simulink model "HSat_orbit_merged_maria"  (R2023b)
settings: Solver=FixedStepAuto  StartTime=0  StopTime=86400*900  MaxStep=3600  RelTol=1e-3  EnableMultiTasking=on
values from neighbouring files (symbols this model uses):
  alpha_acc = sqrt(0.7)    [HSat_op_setup_merged_maria.m]    (also in init_orbit_analysis_with_drag_loss.m)
  ext_ENV_G = 6.674e-11    [HSat_op_setup.m]    (also in HSat_op_setup_merged_maria.m)
  ext_ENV_muEarth = 3.986005e14    (= 398600500000000)    [GEO_insertion_setup.m]    (also in HSat_op_setup.m; HSat_op_setup_merged_maria.m; init_orbit_analysis_with_drag_loss.m)
  ext_ENV_Re = 6.37813700*10^6    (= 6378137)    [HSat_op_setup.m]    (also in HSat_op_setup_merged_maria.m)
  ext_EOR_atmosphere_end = 1000e3    (= 1000000)    [HSat_op_setup.m]    (also in HSat_op_setup_merged_maria.m)
  ext_EOR_perigeeraise_end = 600e3    (= 600000)    [HSat_op_setup.m]    (also in HSat_op_setup_merged_maria.m)
  ext_Main_initDate_IC_T = sim_start    [HSat_op_setup.m]    (also in HSat_op_setup_merged_maria.m)
  ext_SC_activecorr_COE_ECI = [1, 1, 1, 0, 0, 0, 0, 0 ]    [HSat_op_setup.m]    (also in HSat_op_setup_merged_maria.m)
  ext_SC_balanced_COE_ECI = [ .500    0.70    1.100 1 1]    [HSat_op_setup.m]    (also in HSat_op_setup_merged_maria.m = [ 0.10 2.10 1.40    1.0000    1.0000]; launch_settings.m)
  ext_SC_cutofferror_COE_ECI = [150e3, .01, 0.1*pi/180, .1*pi/180,.1*pi/180, 0, 0, 0]    [HSat_op_setup.m]    (also in HSat_op_setup_merged_maria.m)
  ext_SC_init_COE_ECI = [a0,ecc0,i0,an0,ap0,tran0,eccan0,ma0]    [HSat_op_setup.m]    (also in HSat_op_setup_merged_maria.m)
  ext_SC_target_COE_ECI = [a1,ecc1,i1,an1,ap1,tran1,eccan1,ma1]    [HSat_op_setup.m]    (also in HSat_op_setup_merged_maria.m)
  ext_SC_target_lambda = 67*pi/180    (= 1.16937059884)    [HSat_op_setup.m]    (also in HSat_op_setup_merged_maria.m)
  flip_timer = 2*60*60    (= 7200)    [HSat_op_setup_merged_maria.m]
  P_solar = 4.56e-6    (= 4.56e-06)    [HSat_op_setup_merged_maria.m]    (also in init_orbit_analysis_with_drag_loss.m)
  sim_SC_init_CoG_EOR_dry = [-0.00448 0.00106 0.46931]    [HSat_op_setup.m]    (also in HSat_op_setup_merged_maria.m)
  sim_SC_init_CoG_propellant = [0 0 0.24758]    [HSat_op_setup.m]    (also in HSat_op_setup_merged_maria.m)
  sim_SC_init_dry_mass = sim_SC_init_wet_mass-sim_SC_init_propellant_mass    (= 727)    [HSat_op_setup.m]    (also in HSat_op_setup_merged_maria.m = 813.7)
  sim_SC_init_MoI_EOR_wet = [ ... (first row only)    [HSat_op_setup.m]    (also in HSat_op_setup_merged_maria.m; init_orbit_analysis_with_drag_loss.m)
  sim_SC_init_wet_mass = 750    [HSat_op_setup.m]    (also in HSat_op_setup_merged_maria.m)
  sim_thrust_force = [ ... (first row only)    [HSat_op_setup.m]    (also in HSat_op_setup_merged_maria.m)
  sim_thrust_massflow = [ ... (first row only)    [HSat_op_setup.m]    (also in HSat_op_setup_merged_maria.m)
  sim_thrust_vector = [ ... (first row only)    [HSat_op_setup.m]    (also in HSat_op_setup_merged_maria.m)
  sim_thruster_position = [ ... (first row only)    [HSat_op_setup.m]    (also in HSat_op_setup_merged_maria.m)
  sim_ts_save = 60    [HSat_op_setup.m]    (also in HSat_op_setup_merged_maria.m)
  sun_pointing_SA = 0    [HSat_op_setup_merged_maria.m]    (also in init_orbit_analysis_with_drag_loss.m)
  third_body_jupiter = 1    [HSat_op_setup.m]    (also in HSat_op_setup_merged_maria.m)
  third_body_moon = 1    [HSat_op_setup.m]    (also in HSat_op_setup_merged_maria.m)
  third_body_sun = 1    [HSat_op_setup.m]    (also in HSat_op_setup_merged_maria.m)
libraries: aerolibutil x59, simulink x18, matrix_library x16, Toolbox x10, sharedtransform x9, sharedutil x5, aerolibatmos2 x1, simulink_extras x1
(part 5 of 8)

== system HSat_orbit_merged_maria/Subsystem1/control/EORattitude/Subsystem4/Attitude for OR thrusters/Subsystem ==
  EORthrustSCB : Inport
  Create 3x3 Matrix : sharedutil/Create 3x3 Matrix  aMode=aMode
      settings: LibrarySourceBlock=aerolibutil/Create 3x3 Matrix
  Demux : Demux  Outputs=3
  Demux1 : Demux  Outputs=3
  Demux2 : Demux  Outputs=3
  Direction Cosine Matrix to Quaternions : sharedtransform/Direction Cosine Matrix  to Quaternions  aMode=0  action=None  tolerance=eps(2)
      settings: LibrarySourceBlock=|
      | aerolibtransform2/Direction Cosine Matrix
      | to Quaternions
  Quaternion Inverse : aerolibutil/Quaternion Inverse
  VecNormalize4 : Subsystem
      mask Display: disp('u/||u||')
  Zeci x Reci : Subsystem  mask(Cross Product){}
      mask help: Calculates the cross product of two 3x1 vectors.
      mask Help:
      | <p>This block calculates the cross product of two 3x1 vectors, ie.</p>
      | 
      | <ul>C(1) = A(2)*B(3) - A(3)*B(2)</ul>
      | <ul>C(2) = A(3)*B(1) - A(1)*B(3)</ul>
      | <ul>C(3) = A(1)*B(2) - A(2)*B(1)</ul>
      | 
      | <p>The block inputs and output contain more than one signal as described below.</p>
      | 
      | <p><H4>Block Vector Input 1 - A</H4>
      | <ul>
      | <li>A(1)</li>
      | <li>A(2)</li>
      | <li>A(3)</li>
      | </ul>
      | </p>
      | 
      | <p><H4>Block Vector Input 2 - B</H4>
      | <ul>
      | <li>B(1)</li>
      | <li>B(2)</li>
      | <li>B(3)</li>
      | </ul>
      | </p>
      | 
      | <p><H4>Block Vector Output - Cross Product (AxB)</H4>
      | <ul>
      | <li>C(1)</li>
      | <li>C(2)</li>
      | <li>C(3)</li>
      | </ul>
      | </p>
      mask Display: disp('Cross\nProduct')
  Zeci x Reci1 : Subsystem  mask(Cross Product){}
      mask help: Calculates the cross product of two 3x1 vectors.
      mask Help:
      | <p>This block calculates the cross product of two 3x1 vectors, ie.</p>
      | 
      | <ul>C(1) = A(2)*B(3) - A(3)*B(2)</ul>
      | <ul>C(2) = A(3)*B(1) - A(1)*B(3)</ul>
      | <ul>C(3) = A(1)*B(2) - A(2)*B(1)</ul>
      | 
      | <p>The block inputs and output contain more than one signal as described below.</p>
      | 
      | <p><H4>Block Vector Input 1 - A</H4>
      | <ul>
      | <li>A(1)</li>
      | <li>A(2)</li>
      | <li>A(3)</li>
      | </ul>
      | </p>
      | 
      | <p><H4>Block Vector Input 2 - B</H4>
      | <ul>
      | <li>B(1)</li>
      | <li>B(2)</li>
      | <li>B(3)</li>
      | </ul>
      | </p>
      | 
      | <p><H4>Block Vector Output - Cross Product (AxB)</H4>
      | <ul>
      | <li>C(1)</li>
      | <li>C(2)</li>
      | <li>C(3)</li>
      | </ul>
      | </p>
      mask Display: disp('Cross\nProduct')
  yscbSCB : Constant  Value=[0 1 0]
  qscbp2scb : Outport
  wires:
  Direction Cosine Matrix to Quaternions/1 -> Quaternion Inverse/1  "qscbp2scb"
  Demux2/3 -> Create 3x3 Matrix/9
  Demux2/1 -> Create 3x3 Matrix/7
  Demux/1 -> Create 3x3 Matrix/1
  Demux1/2 -> Create 3x3 Matrix/5
  EORthrustSCB/1 -> VecNormalize4/1(In1)
  Demux2/2 -> Create 3x3 Matrix/8
  Demux/3 -> Create 3x3 Matrix/3
  Zeci x Reci/1(c(1) c(2) c(3)) -> Zeci x Reci1/2(b(1) b(2) b(3)), Demux/1  "xscbpSCB"
  Demux/2 -> Create 3x3 Matrix/2
  Create 3x3 Matrix/1 -> Direction Cosine Matrix to Quaternions/1
  Zeci x Reci1/1(c(1) c(2) c(3)) -> Demux1/1  "yscbpSCB"
  Demux1/3 -> Create 3x3 Matrix/6
  Demux1/1 -> Create 3x3 Matrix/4
  yscbSCB/1 -> Zeci x Reci/1(a(1) a(2) a(3))
  VecNormalize4/1(Out1) -> Demux2/1, Zeci x Reci1/1(a(1) a(2) a(3)), Zeci x Reci/2(b(1) b(2) b(3))  "zscbpSCB"
  Quaternion Inverse/1 -> qscbp2scb/1

== system HSat_orbit_merged_maria/Subsystem1/control/EORattitude/Subsystem4/Attitude for OR thrusters/q_scb_calc ==
  EORthrustECI : Inport
  sunvECI : Inport  Port=2
  Direction Cosine Matrix to Quaternions : sharedtransform/Direction Cosine Matrix  to Quaternions  aMode=0  action=None  tolerance=eps(2)
      settings: LibrarySourceBlock=|
      | aerolibtransform2/Direction Cosine Matrix
      | to Quaternions
  Matrix Concatenate : Concatenate  NumInputs=3  Mode=Multidimensional array
  Reshape1 : Reshape  OutputDimensionality=Row vector (2-D)
  Reshape2 : Reshape  OutputDimensionality=Row vector (2-D)
  Reshape3 : Reshape  OutputDimensionality=Row vector (2-D)
  VecNormalize : Subsystem
      mask Display: disp('u/||u||')
  VecNormalize1 : Subsystem
      mask Display: disp('u/||u||')
  VecNormalize2 : Subsystem
      mask Display: disp('u/||u||')
  VecNormalize3 : Subsystem
      mask Display: disp('u/||u||')
  Yscb x Zscb : Subsystem  mask(Cross Product){}
      mask help: Calculates the cross product of two 3x1 vectors.
      mask Help:
      | <p>This block calculates the cross product of two 3x1 vectors, ie.</p>
      | 
      | <ul>C(1) = A(2)*B(3) - A(3)*B(2)</ul>
      | <ul>C(2) = A(3)*B(1) - A(1)*B(3)</ul>
      | <ul>C(3) = A(1)*B(2) - A(2)*B(1)</ul>
      | 
      | <p>The block inputs and output contain more than one signal as described below.</p>
      | 
      | <p><H4>Block Vector Input 1 - A</H4>
      | <ul>
      | <li>A(1)</li>
      | <li>A(2)</li>
      | <li>A(3)</li>
      | </ul>
      | </p>
      | 
      | <p><H4>Block Vector Input 2 - B</H4>
      | <ul>
      | <li>B(1)</li>
      | <li>B(2)</li>
      | <li>B(3)</li>
      | </ul>
      | </p>
      | 
      | <p><H4>Block Vector Output - Cross Product (AxB)</H4>
      | <ul>
      | <li>C(1)</li>
      | <li>C(2)</li>
      | <li>C(3)</li>
      | </ul>
      | </p>
      mask Display: disp('Cross\nProduct')
  Zeci x Reci : Subsystem  mask(Cross Product){}
      mask help: Calculates the cross product of two 3x1 vectors.
      mask Help:
      | <p>This block calculates the cross product of two 3x1 vectors, ie.</p>
      | 
      | <ul>C(1) = A(2)*B(3) - A(3)*B(2)</ul>
      | <ul>C(2) = A(3)*B(1) - A(1)*B(3)</ul>
      | <ul>C(3) = A(1)*B(2) - A(2)*B(1)</ul>
      | 
      | <p>The block inputs and output contain more than one signal as described below.</p>
      | 
      | <p><H4>Block Vector Input 1 - A</H4>
      | <ul>
      | <li>A(1)</li>
      | <li>A(2)</li>
      | <li>A(3)</li>
      | </ul>
      | </p>
      | 
      | <p><H4>Block Vector Input 2 - B</H4>
      | <ul>
      | <li>B(1)</li>
      | <li>B(2)</li>
      | <li>B(3)</li>
      | </ul>
      | </p>
      | 
      | <p><H4>Block Vector Output - Cross Product (AxB)</H4>
      | <ul>
      | <li>C(1)</li>
      | <li>C(2)</li>
      | <li>C(3)</li>
      | </ul>
      | </p>
      mask Display: disp('Cross\nProduct')
  qECI2scbp : Outport  InitialOutput=0
  wires:
  Zeci x Reci/1(c(1) c(2) c(3)) -> VecNormalize3/1(In1)  "Y"
  VecNormalize1/1(Out1) -> Yscb x Zscb/2(b(1) b(2) b(3)), Reshape3/1, Zeci x Reci/2(b(1) b(2) b(3))  "Zscbp"
  Direction Cosine Matrix to Quaternions/1 -> qECI2scbp/1
  EORthrustECI/1 -> VecNormalize1/1(In1)
  VecNormalize3/1(Out1) -> Reshape1/1, Yscb x Zscb/1(a(1) a(2) a(3))  "Yscbp"
  Yscb x Zscb/1(c(1) c(2) c(3)) -> VecNormalize/1(In1)
  sunvECI/1 -> VecNormalize2/1(In1)
  Reshape1/1 -> Matrix Concatenate/2
  Reshape3/1 -> Matrix Concatenate/3
  Reshape2/1 -> Matrix Concatenate/1
  VecNormalize/1(Out1) -> Reshape2/1  "Xscbp"
  VecNormalize2/1(Out1) -> Zeci x Reci/1(a(1) a(2) a(3))
  Matrix Concatenate/1 -> Direction Cosine Matrix to Quaternions/1

== system HSat_orbit_merged_maria/Subsystem1/control/EORattitude/Subsystem4/Attitude for SK unloading/Subsystem ==
  SKtorqueSCB : Inport
  Create 3x3 Matrix : sharedutil/Create 3x3 Matrix  aMode=aMode
      settings: LibrarySourceBlock=aerolibutil/Create 3x3 Matrix
  Demux : Demux  Outputs=3
  Demux1 : Demux  Outputs=3
  Demux2 : Demux  Outputs=3
  Direction Cosine Matrix to Quaternions : sharedtransform/Direction Cosine Matrix  to Quaternions  aMode=0  action=None  tolerance=eps(2)
      settings: LibrarySourceBlock=|
      | aerolibtransform2/Direction Cosine Matrix
      | to Quaternions
  Quaternion Inverse : aerolibutil/Quaternion Inverse
  VecNormalize4 : Subsystem
      mask Display: disp('u/||u||')
  Zeci x Reci : Subsystem  mask(Cross Product){}
      mask help: Calculates the cross product of two 3x1 vectors.
      mask Help:
      | <p>This block calculates the cross product of two 3x1 vectors, ie.</p>
      | 
      | <ul>C(1) = A(2)*B(3) - A(3)*B(2)</ul>
      | <ul>C(2) = A(3)*B(1) - A(1)*B(3)</ul>
      | <ul>C(3) = A(1)*B(2) - A(2)*B(1)</ul>
      | 
      | <p>The block inputs and output contain more than one signal as described below.</p>
      | 
      | <p><H4>Block Vector Input 1 - A</H4>
      | <ul>
      | <li>A(1)</li>
      | <li>A(2)</li>
      | <li>A(3)</li>
      | </ul>
      | </p>
      | 
      | <p><H4>Block Vector Input 2 - B</H4>
      | <ul>
      | <li>B(1)</li>
      | <li>B(2)</li>
      | <li>B(3)</li>
      | </ul>
      | </p>
      | 
      | <p><H4>Block Vector Output - Cross Product (AxB)</H4>
      | <ul>
      | <li>C(1)</li>
      | <li>C(2)</li>
      | <li>C(3)</li>
      | </ul>
      | </p>
      mask Display: disp('Cross\nProduct')
  Zeci x Reci1 : Subsystem  mask(Cross Product){}
      mask help: Calculates the cross product of two 3x1 vectors.
      mask Help:
      | <p>This block calculates the cross product of two 3x1 vectors, ie.</p>
      | 
      | <ul>C(1) = A(2)*B(3) - A(3)*B(2)</ul>
      | <ul>C(2) = A(3)*B(1) - A(1)*B(3)</ul>
      | <ul>C(3) = A(1)*B(2) - A(2)*B(1)</ul>
      | 
      | <p>The block inputs and output contain more than one signal as described below.</p>
      | 
      | <p><H4>Block Vector Input 1 - A</H4>
      | <ul>
      | <li>A(1)</li>
      | <li>A(2)</li>
      | <li>A(3)</li>
      | </ul>
      | </p>
      | 
      | <p><H4>Block Vector Input 2 - B</H4>
      | <ul>
      | <li>B(1)</li>
      | <li>B(2)</li>
      | <li>B(3)</li>
      | </ul>
      | </p>
      | 
      | <p><H4>Block Vector Output - Cross Product (AxB)</H4>
      | <ul>
      | <li>C(1)</li>
      | <li>C(2)</li>
      | <li>C(3)</li>
      | </ul>
      | </p>
      mask Display: disp('Cross\nProduct')
  yscbSCB : Constant  Value=[0 1 0]
  qscbp2scb : Outport
  wires:
  Direction Cosine Matrix to Quaternions/1 -> Quaternion Inverse/1  "qscbp2scb"
  Demux2/3 -> Create 3x3 Matrix/9
  Demux2/1 -> Create 3x3 Matrix/7
  Demux/1 -> Create 3x3 Matrix/1
  Demux1/2 -> Create 3x3 Matrix/5
  SKtorqueSCB/1 -> VecNormalize4/1(In1)
  Demux2/2 -> Create 3x3 Matrix/8
  Demux/3 -> Create 3x3 Matrix/3
  Zeci x Reci/1(c(1) c(2) c(3)) -> Zeci x Reci1/2(b(1) b(2) b(3)), Demux/1  "xscbpSCB"
  Demux/2 -> Create 3x3 Matrix/2
  Create 3x3 Matrix/1 -> Direction Cosine Matrix to Quaternions/1
  Zeci x Reci1/1(c(1) c(2) c(3)) -> Demux1/1  "yscbpSCB"
  Demux1/3 -> Create 3x3 Matrix/6
  Demux1/1 -> Create 3x3 Matrix/4
  yscbSCB/1 -> Zeci x Reci/1(a(1) a(2) a(3))
  VecNormalize4/1(Out1) -> Demux2/1, Zeci x Reci1/1(a(1) a(2) a(3)), Zeci x Reci/2(b(1) b(2) b(3))  "zscbpSCB"
  Quaternion Inverse/1 -> qscbp2scb/1

== system HSat_orbit_merged_maria/Subsystem1/control/EORattitude/Subsystem4/Attitude for SK unloading/VecNormalize ==
  In1 : Inport
  Constant : Constant
  Demux : Demux  Outputs=[-1 1]
  Divide : Product  Inputs=*/  OutDataTypeStr=double
  Ground : Ground
  Math Function : Math  Operator=square  SignedPower=on
  Math Function1 : Math  Operator=sqrt  SignedPower=on
  Mux : Mux  Inputs=2
  Mux1 : Mux  Inputs=2
  Product : Product  RndMeth=Zero
  Sum of Elements : Sum  Inputs=+
  Switch : Switch  Criteria=u2 > Threshold  Threshold=eps  SaturateOnIntegerOverflow=off  InputSameDT=off
  Out1 : Outport  VectorParamsAs1DForOutWhenUnconnected=off
  wires:
  Math Function/1 -> Sum of Elements/1
  Demux/1 -> Divide/1
  Constant/1 -> Mux1/2
  Mux1/1 -> Switch/3
  Divide/1 -> Out1/1
  Switch/1 -> Demux/1
  Mux/1 -> Switch/1
  Demux/2 -> Divide/2
  Product/1 -> Mux1/1
  In1/1 -> Product/1, Math Function/1, Mux/1
  Ground/1 -> Product/2
  Sum of Elements/1 -> Math Function1/1
  Math Function1/1 -> Mux/2, Switch/2

== system HSat_orbit_merged_maria/Subsystem1/control/EORattitude/Subsystem4/Attitude for SK unloading/VecNormalize1 ==
  In1 : Inport
  Constant : Constant
  Demux : Demux  Outputs=[-1 1]
  Divide : Product  Inputs=*/  OutDataTypeStr=double
  Ground : Ground
  Math Function : Math  Operator=square  SignedPower=on
  Math Function1 : Math  Operator=sqrt  SignedPower=on
  Mux : Mux  Inputs=2
  Mux1 : Mux  Inputs=2
  Product : Product  RndMeth=Zero
  Sum of Elements : Sum  Inputs=+
  Switch : Switch  Criteria=u2 > Threshold  Threshold=eps  SaturateOnIntegerOverflow=off  InputSameDT=off
  Out1 : Outport  VectorParamsAs1DForOutWhenUnconnected=off
  wires:
  Math Function/1 -> Sum of Elements/1
  Demux/1 -> Divide/1
  Constant/1 -> Mux1/2
  Mux1/1 -> Switch/3
  Divide/1 -> Out1/1
  Switch/1 -> Demux/1
  Mux/1 -> Switch/1
  Demux/2 -> Divide/2
  Product/1 -> Mux1/1
  In1/1 -> Product/1, Math Function/1, Mux/1
  Ground/1 -> Product/2
  Sum of Elements/1 -> Math Function1/1
  Math Function1/1 -> Mux/2, Switch/2

== system HSat_orbit_merged_maria/Subsystem1/control/EORattitude/Subsystem4/Attitude for SK unloading/VecNormalize2 ==
  In1 : Inport
  Constant : Constant
  Demux : Demux  Outputs=[-1 1]
  Divide : Product  Inputs=*/  OutDataTypeStr=double
  Ground : Ground
  Math Function : Math  Operator=square  SignedPower=on
  Math Function1 : Math  Operator=sqrt  SignedPower=on
  Mux : Mux  Inputs=2
  Mux1 : Mux  Inputs=2
  Product : Product  RndMeth=Zero
  Sum of Elements : Sum  Inputs=+
  Switch : Switch  Criteria=u2 > Threshold  Threshold=eps  SaturateOnIntegerOverflow=off  InputSameDT=off
  Out1 : Outport  VectorParamsAs1DForOutWhenUnconnected=off
  wires:
  Math Function/1 -> Sum of Elements/1
  Demux/1 -> Divide/1
  Constant/1 -> Mux1/2
  Mux1/1 -> Switch/3
  Divide/1 -> Out1/1
  Switch/1 -> Demux/1
  Mux/1 -> Switch/1
  Demux/2 -> Divide/2
  Product/1 -> Mux1/1
  In1/1 -> Product/1, Math Function/1, Mux/1
  Ground/1 -> Product/2
  Sum of Elements/1 -> Math Function1/1
  Math Function1/1 -> Mux/2, Switch/2

== system HSat_orbit_merged_maria/Subsystem1/control/EORattitude/Subsystem4/Attitude for SK unloading/VecNormalize3 ==
  In1 : Inport
  Constant : Constant
  Demux : Demux  Outputs=[-1 1]
  Divide : Product  Inputs=*/  OutDataTypeStr=double
  Ground : Ground
  Math Function : Math  Operator=square  SignedPower=on
  Math Function1 : Math  Operator=sqrt  SignedPower=on
  Mux : Mux  Inputs=2
  Mux1 : Mux  Inputs=2
  Product : Product  RndMeth=Zero
  Sum of Elements : Sum  Inputs=+
  Switch : Switch  Criteria=u2 > Threshold  Threshold=eps  SaturateOnIntegerOverflow=off  InputSameDT=off
  Out1 : Outport  VectorParamsAs1DForOutWhenUnconnected=off
  wires:
  Math Function/1 -> Sum of Elements/1
  Demux/1 -> Divide/1
  Constant/1 -> Mux1/2
  Mux1/1 -> Switch/3
  Divide/1 -> Out1/1
  Switch/1 -> Demux/1
  Mux/1 -> Switch/1
  Demux/2 -> Divide/2
  Product/1 -> Mux1/1
  In1/1 -> Product/1, Math Function/1, Mux/1
  Ground/1 -> Product/2
  Sum of Elements/1 -> Math Function1/1
  Math Function1/1 -> Mux/2, Switch/2

== system HSat_orbit_merged_maria/Subsystem1/control/EORattitude/Subsystem4/Attitude for SK unloading/Yscb x Zscb ==
  a(1) a(2) a(3) : Inport
  b(1) b(2) b(3) : Inport  Port=2
  Product : Product  InputSameDT=on  SaturateOnIntegerOverflow=on  OutDataTypeStr=Inherit: Same as first input
  Product1 : Product  InputSameDT=on  SaturateOnIntegerOverflow=on  OutDataTypeStr=Inherit: Same as first input
  Selector : Selector  InputPortWidth=3  IndexOptions=Index vector (dialog)  Indices=[2 3 1]  OutputSizes=1
  Selector1 : Selector  InputPortWidth=3  IndexOptions=Index vector (dialog)  Indices=[3 1 2]  OutputSizes=1
  Selector2 : Selector  InputPortWidth=3  IndexOptions=Index vector (dialog)  Indices=[2 3 1]  OutputSizes=1
  Selector3 : Selector  InputPortWidth=3  IndexOptions=Index vector (dialog)  Indices=[3 1 2]  OutputSizes=1
  Sum : Sum  Inputs=+|-  InputSameDT=on  SaturateOnIntegerOverflow=on  OutDataTypeStr=Inherit: Same as first input
  c(1) c(2) c(3) : Outport  InitialOutput=0
  wires:
  Sum/1 -> c(1) c(2) c(3)/1
  b(1) b(2) b(3)/1 -> Selector1/1, Selector2/1
  Selector/1 -> Product/1
  a(1) a(2) a(3)/1 -> Selector/1, Selector3/1
  Product/1 -> Sum/1
  Selector1/1 -> Product/2
  Product1/1 -> Sum/2
  Selector2/1 -> Product1/2
  Selector3/1 -> Product1/1

== system HSat_orbit_merged_maria/Subsystem1/control/EORattitude/Subsystem4/Attitude for SK unloading/Zeci x Reci ==
  a(1) a(2) a(3) : Inport
  b(1) b(2) b(3) : Inport  Port=2
  Product : Product  InputSameDT=on  SaturateOnIntegerOverflow=on  OutDataTypeStr=Inherit: Same as first input
  Product1 : Product  InputSameDT=on  SaturateOnIntegerOverflow=on  OutDataTypeStr=Inherit: Same as first input
  Selector : Selector  InputPortWidth=3  IndexOptions=Index vector (dialog)  Indices=[2 3 1]  OutputSizes=1
  Selector1 : Selector  InputPortWidth=3  IndexOptions=Index vector (dialog)  Indices=[3 1 2]  OutputSizes=1
  Selector2 : Selector  InputPortWidth=3  IndexOptions=Index vector (dialog)  Indices=[2 3 1]  OutputSizes=1
  Selector3 : Selector  InputPortWidth=3  IndexOptions=Index vector (dialog)  Indices=[3 1 2]  OutputSizes=1
  Sum : Sum  Inputs=+|-  InputSameDT=on  SaturateOnIntegerOverflow=on  OutDataTypeStr=Inherit: Same as first input
  c(1) c(2) c(3) : Outport  InitialOutput=0
  wires:
  Selector3/1 -> Product1/1
  Selector2/1 -> Product1/2
  Product1/1 -> Sum/2
  Selector1/1 -> Product/2
  Product/1 -> Sum/1
  a(1) a(2) a(3)/1 -> Selector3/1, Selector/1
  Selector/1 -> Product/1
  b(1) b(2) b(3)/1 -> Selector2/1, Selector1/1
  Sum/1 -> c(1) c(2) c(3)/1

== system HSat_orbit_merged_maria/Subsystem1/control/EORattitude/Subsystem4/Subsystem3/Flip satellite based on worst case faior ==
  AmomSCB : Inport
  thrustscb : Inport  Port=2
  Constant : Constant  Value=sim_SC_init_MoI_EOR_wet
  MATLAB Function : MATLAB Function  TreatAsAtomicUnit=on
  Reshape : Reshape  OutputDimensionality=Column vector (2-D)
  Scope : Scope  NumInputPorts=2
  worstRwMom : Outport
  isFlip : Outport  Port=2
  idxMinMom : Outport  Port=3
  wires:
  AmomSCB/1 -> Reshape/1
  thrustscb/1 -> MATLAB Function/2(thrustVect)
  MATLAB Function/1(worstRwMom) -> Scope/1, worstRwMom/1  "worstRwmom"
  MATLAB Function/2(isFlip) -> Scope/2, isFlip/1  "flip"
  MATLAB Function/3(idxMaxMom) -> idxMinMom/1
  Constant/1 -> MATLAB Function/3(scInertia)
  Reshape/1 -> MATLAB Function/1(scMom)

== system HSat_orbit_merged_maria/Subsystem1/control/EORattitude/Subsystem4/Subsystem3/FlipSatellite ==
  AmomSCB : Inport
  EORtorqueSCB : Inport  Port=2
  Compare To Constant : simulink/Logic and Bit Operations/Compare To Constant  relop=>  const=sin((180-70.53)/2*pi/180)*25*.75  OutDataTypeStr=boolean
  Compare To Constant1 : simulink/Logic and Bit Operations/Compare To Constant  relop=>  const=cos(80*pi/180)  OutDataTypeStr=boolean
  Compare To Constant2 : simulink/Logic and Bit Operations/Compare To Constant  relop=>  const=sin((180-70.53)/2*pi/180)*25*.8  OutDataTypeStr=boolean
  Compare To Constant3 : simulink/Logic and Bit Operations/Compare To Constant  relop=>  const=cos(90*pi/180)  OutDataTypeStr=boolean
  Dot Product : DotProduct  OutDataTypeStr=Inherit: Inherit via internal rule
  Dot Product1 : DotProduct  OutDataTypeStr=Inherit: Inherit via internal rule
  Logical Operator : Logic  AllPortsSameDT=off  OutDataTypeStr=boolean
  Logical Operator1 : Logic  AllPortsSameDT=off  OutDataTypeStr=boolean
  Logical Operator2 : Logic  Operator=OR  AllPortsSameDT=off  OutDataTypeStr=boolean
  Logical Operator3 : Logic  Operator=NOT  AllPortsSameDT=off  OutDataTypeStr=boolean
  Reshape1 : Reshape  OutputDimensionality=Row vector (2-D)
  VecNormalize : Subsystem
      mask Display: disp('u/||u||')
  VecNormalize1 : Subsystem
      mask Display: disp('u/||u||')
  FlipSatellite_bool : Outport
  DoAMOM : Outport  Port=2
  NoAMOM : Outport  Port=3
  wires:
  Logical Operator/1 -> Logical Operator2/1
  EORtorqueSCB/1 -> VecNormalize1/1(In1)
  Dot Product/1 -> Compare To Constant2/1, Compare To Constant/1
  Compare To Constant/1 -> Logical Operator/1
  Dot Product1/1 -> Compare To Constant3/1, Compare To Constant1/1
  Compare To Constant1/1 -> Logical Operator/2
  VecNormalize/1(Out1) -> Dot Product/2, Dot Product1/1
  VecNormalize1/1(Out1) -> Dot Product1/2
  Compare To Constant2/1 -> Logical Operator1/1
  Compare To Constant3/1 -> Logical Operator3/1, Logical Operator1/2
  Logical Operator1/1 -> DoAMOM/1, Logical Operator2/2
  Logical Operator2/1 -> FlipSatellite_bool/1
  AmomSCB/1 -> Reshape1/1
  Reshape1/1 -> Dot Product/1, VecNormalize/1(In1)
  Logical Operator3/1 -> NoAMOM/1

== system HSat_orbit_merged_maria/Subsystem1/control/EORattitude/Subsystem4/Subsystem3/Subsystem ==
  note: When FlipNow = 1, FlipPlusMinus changes
      | from 0 -> 1 or 1 -> 0.
      | When FlipNow  = 0, FlipPlusMinus keeps the
      | value it has.
  note: FlipSign
  FlipNow : Inport
  Logical Operator : Logic  Operator=NOT  AllPortsSameDT=off  OutDataTypeStr=boolean
  Switch : Switch  Criteria=u2 > Threshold  SaturateOnIntegerOverflow=off
  Unit Delay : UnitDelay  InitialCondition=false  SampleTime=-1  HasFrameUpgradeWarning=on
  FlipPlusMinus : Outport
  wires:
  FlipNow/1 -> Switch/2
  Logical Operator/1 -> Switch/1
  Switch/1 -> Unit Delay/1, FlipPlusMinus/1
  Unit Delay/1 -> Logical Operator/1, Switch/3

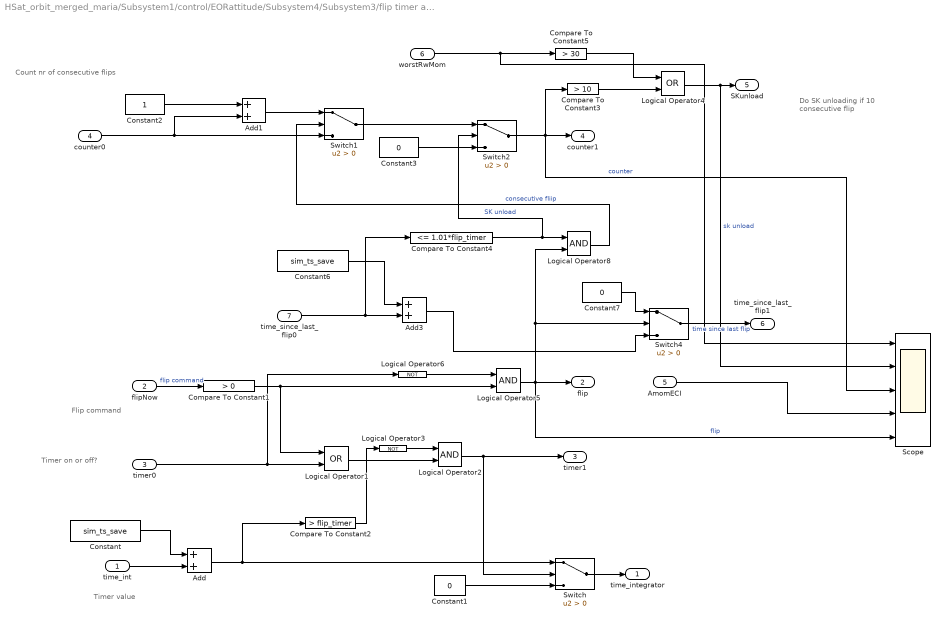
== system HSat_orbit_merged_maria/Subsystem1/control/EORattitude/Subsystem4/Subsystem3/flip timer and SK trigger ==
  note: Timer on or off?
  note: Flip command
  note: Timer value
  note: Count nr of
      | consecutive flips
  note: Do SK unloading
      | if 10 consecutive
      | flip
  time_int : Inport
  flipNow : Inport  Port=2
  timer0 : Inport  Port=3
  counter0 : Inport  Port=4
  AmomECI : Inport  Port=5
  worstRwMom : Inport  Port=6
  time_since_last_flip0 : Inport  Port=7
  Add : Sum
  Add1 : Sum
  Add3 : Sum
  Compare To Constant1 : simulink/Logic and Bit Operations/Compare To Constant  relop=>  const=0  OutDataTypeStr=boolean
  Compare To Constant2 : simulink/Logic and Bit Operations/Compare To Constant  relop=>  const=flip_timer  OutDataTypeStr=boolean
  Compare To Constant3 : simulink/Logic and Bit Operations/Compare To Constant  relop=>  const=10  OutDataTypeStr=boolean
  Compare To Constant4 : simulink/Logic and Bit Operations/Compare To Constant  relop=<=  const=1.01*flip_timer  OutDataTypeStr=boolean
  Compare To Constant5 : simulink/Logic and Bit Operations/Compare To Constant  relop=>  const=30  OutDataTypeStr=boolean
  Constant : Constant  Value=sim_ts_save
  Constant1 : Constant  Value=0
  Constant2 : Constant
  Constant3 : Constant  Value=0
  Constant6 : Constant  Value=sim_ts_save
  Constant7 : Constant  Value=0
  Logical Operator1 : Logic  Operator=OR  AllPortsSameDT=off  OutDataTypeStr=boolean
  Logical Operator2 : Logic  AllPortsSameDT=off  OutDataTypeStr=boolean
  Logical Operator3 : Logic  Operator=NOT  AllPortsSameDT=off  OutDataTypeStr=boolean
  Logical Operator4 : Logic  Operator=OR  AllPortsSameDT=off  OutDataTypeStr=boolean
  Logical Operator5 : Logic  AllPortsSameDT=off  OutDataTypeStr=boolean
  Logical Operator6 : Logic  Operator=NOT  AllPortsSameDT=off  OutDataTypeStr=boolean
  Logical Operator8 : Logic  AllPortsSameDT=off  OutDataTypeStr=boolean
  Scope : Scope  NumInputPorts=5
  Switch{,1..2,4} (4 alike) : Switch  Criteria=u2 > Threshold  SaturateOnIntegerOverflow=off  InputSameDT=off
  time_integrator : Outport
  flip : Outport  Port=2
  timer1 : Outport  Port=3
  counter1 : Outport  Port=4
  SKunload : Outport  Port=5
  time_since_last_flip1 : Outport  Port=6
  wires:
  flipNow/1 -> Compare To Constant1/1  "flip command"
  time_int/1 -> Add/2
  Constant/1 -> Add/1
  Add/1 -> Switch/1, Compare To Constant2/1
  Compare To Constant1/1 -> Logical Operator5/2, Logical Operator1/1
  Compare To Constant2/1 -> Logical Operator3/1
  Logical Operator5/1 -> Switch4/2, Logical Operator8/2, flip/1, Scope/5  "flip"
  Switch/1 -> time_integrator/1
  Constant1/1 -> Switch/3
  Logical Operator1/1 -> Logical Operator2/2
  Logical Operator3/1 -> Logical Operator2/1
  Logical Operator2/1 -> timer1/1, Switch/2
  counter0/1 -> Add1/2, Switch1/3
  Constant2/1 -> Add1/1
  Add1/1 -> Switch1/1
  Switch1/1 -> Switch2/1
  timer0/1 -> Logical Operator6/1, Logical Operator1/2
  Constant3/1 -> Switch2/3
  Switch2/1 -> Scope/3, Compare To Constant3/1, counter1/1  "counter"
  Logical Operator6/1 -> Logical Operator5/1
  AmomECI/1 -> Scope/4
  worstRwMom/1 -> Scope/1, Compare To Constant5/1
  Constant6/1 -> Add3/1
  Add3/1 -> Switch4/3
  Constant7/1 -> Switch4/1
  Switch4/1 -> time_since_last_flip1/1  "time since last flip"
  Compare To Constant4/1 -> Switch2/2, Logical Operator8/1  "SK unload"
  time_since_last_flip0/1 -> Compare To Constant4/1, Add3/2
  Logical Operator8/1 -> Switch1/2  "consecutive fliip"
  Compare To Constant3/1 -> Logical Operator4/2
  Logical Operator4/1 -> Scope/2, SKunload/1  "sk unload"
  Compare To Constant5/1 -> Logical Operator4/1

== system HSat_orbit_merged_maria/Subsystem1/control/EORattitude/Subsystem4/flips around thrust vector/VecNormalize4 ==
  In1 : Inport
  Constant : Constant
  Demux : Demux  Outputs=[-1 1]
  Divide : Product  Inputs=*/  OutDataTypeStr=double
  Ground : Ground
  Math Function : Math  Operator=square  SignedPower=on
  Math Function1 : Math  Operator=sqrt  SignedPower=on
  Mux : Mux  Inputs=2
  Mux1 : Mux  Inputs=2
  Product : Product  RndMeth=Zero
  Sum of Elements : Sum  Inputs=+
  Switch : Switch  Criteria=u2 > Threshold  Threshold=eps  SaturateOnIntegerOverflow=off  InputSameDT=off
  Out1 : Outport  VectorParamsAs1DForOutWhenUnconnected=off
  wires:
  Math Function/1 -> Sum of Elements/1
  Demux/1 -> Divide/1
  Constant/1 -> Mux1/2
  Mux1/1 -> Switch/3
  Divide/1 -> Out1/1
  Switch/1 -> Demux/1
  Mux/1 -> Switch/1
  Demux/2 -> Divide/2
  Product/1 -> Mux1/1
  In1/1 -> Product/1, Math Function/1, Mux/1
  Ground/1 -> Product/2
  Sum of Elements/1 -> Math Function1/1
  Math Function1/1 -> Mux/2, Switch/2

== system HSat_orbit_merged_maria/Subsystem1/control/Subsystem6/Subsystem2/PPU1/VecNormalize1 ==
  In1 : Inport
  Constant : Constant
  Demux : Demux  Outputs=[-1 1]
  Divide : Product  Inputs=*/  OutDataTypeStr=double
  Ground : Ground
  Math Function : Math  Operator=square  SignedPower=on
  Math Function1 : Math  Operator=sqrt  SignedPower=on
  Mux : Mux  Inputs=2
  Mux1 : Mux  Inputs=2
  Product : Product  RndMeth=Zero
  Sum of Elements : Sum  Inputs=+
  Switch : Switch  Criteria=u2 > Threshold  Threshold=eps  SaturateOnIntegerOverflow=off  InputSameDT=off
  Out1 : Outport  VectorParamsAs1DForOutWhenUnconnected=off
  wires:
  Math Function/1 -> Sum of Elements/1
  Demux/1 -> Divide/1
  Constant/1 -> Mux1/2
  Mux1/1 -> Switch/3
  Divide/1 -> Out1/1
  Switch/1 -> Demux/1
  Mux/1 -> Switch/1
  Demux/2 -> Divide/2
  Product/1 -> Mux1/1
  In1/1 -> Product/1, Math Function/1, Mux/1
  Ground/1 -> Product/2
  Sum of Elements/1 -> Math Function1/1
  Math Function1/1 -> Mux/2, Switch/2

== system HSat_orbit_merged_maria/Subsystem1/control/Subsystem6/Subsystem2/PPU1/VecNormalize2 ==
  In1 : Inport
  Constant : Constant
  Demux : Demux  Outputs=[-1 1]
  Divide : Product  Inputs=*/  OutDataTypeStr=double
  Ground : Ground
  Math Function : Math  Operator=square  SignedPower=on
  Math Function1 : Math  Operator=sqrt  SignedPower=on
  Mux : Mux  Inputs=2
  Mux1 : Mux  Inputs=2
  Product : Product  RndMeth=Zero
  Sum of Elements : Sum  Inputs=+
  Switch : Switch  Criteria=u2 > Threshold  Threshold=eps  SaturateOnIntegerOverflow=off  InputSameDT=off
  Out1 : Outport  VectorParamsAs1DForOutWhenUnconnected=off
  wires:
  Math Function/1 -> Sum of Elements/1
  Demux/1 -> Divide/1
  Constant/1 -> Mux1/2
  Mux1/1 -> Switch/3
  Divide/1 -> Out1/1
  Switch/1 -> Demux/1
  Mux/1 -> Switch/1
  Demux/2 -> Divide/2
  Product/1 -> Mux1/1
  In1/1 -> Product/1, Math Function/1, Mux/1
  Ground/1 -> Product/2
  Sum of Elements/1 -> Math Function1/1
  Math Function1/1 -> Mux/2, Switch/2

== system HSat_orbit_merged_maria/Subsystem1/control/Subsystem6/Subsystem2/PPU1/VecNormalize3 ==
  In1 : Inport
  Constant : Constant
  Demux : Demux  Outputs=[-1 1]
  Divide : Product  Inputs=*/  OutDataTypeStr=double
  Ground : Ground
  Math Function : Math  Operator=square  SignedPower=on
  Math Function1 : Math  Operator=sqrt  SignedPower=on
  Mux : Mux  Inputs=2
  Mux1 : Mux  Inputs=2
  Product : Product  RndMeth=Zero
  Sum of Elements : Sum  Inputs=+
  Switch : Switch  Criteria=u2 > Threshold  Threshold=eps  SaturateOnIntegerOverflow=off  InputSameDT=off
  Out1 : Outport  VectorParamsAs1DForOutWhenUnconnected=off
  wires:
  Math Function/1 -> Sum of Elements/1
  Demux/1 -> Divide/1
  Constant/1 -> Mux1/2
  Mux1/1 -> Switch/3
  Divide/1 -> Out1/1
  Switch/1 -> Demux/1
  Mux/1 -> Switch/1
  Demux/2 -> Divide/2
  Product/1 -> Mux1/1
  In1/1 -> Product/1, Math Function/1, Mux/1
  Ground/1 -> Product/2
  Sum of Elements/1 -> Math Function1/1
  Math Function1/1 -> Mux/2, Switch/2

== system HSat_orbit_merged_maria/Subsystem1/control/Subsystem6/Subsystem2/PPU1/VecNormalize4 ==
  In1 : Inport
  Constant : Constant
  Demux : Demux  Outputs=[-1 1]
  Divide : Product  Inputs=*/  OutDataTypeStr=double
  Ground : Ground
  Math Function : Math  Operator=square  SignedPower=on
  Math Function1 : Math  Operator=sqrt  SignedPower=on
  Mux : Mux  Inputs=2
  Mux1 : Mux  Inputs=2
  Product : Product  RndMeth=Zero
  Sum of Elements : Sum  Inputs=+
  Switch : Switch  Criteria=u2 > Threshold  Threshold=eps  SaturateOnIntegerOverflow=off  InputSameDT=off
  Out1 : Outport  VectorParamsAs1DForOutWhenUnconnected=off
  wires:
  Math Function/1 -> Sum of Elements/1
  Demux/1 -> Divide/1
  Constant/1 -> Mux1/2
  Mux1/1 -> Switch/3
  Divide/1 -> Out1/1
  Switch/1 -> Demux/1
  Mux/1 -> Switch/1
  Demux/2 -> Divide/2
  Product/1 -> Mux1/1
  In1/1 -> Product/1, Math Function/1, Mux/1
  Ground/1 -> Product/2
  Sum of Elements/1 -> Math Function1/1
  Math Function1/1 -> Mux/2, Switch/2

== system HSat_orbit_merged_maria/Subsystem1/control/Subsystem6/Subsystem2/PPU1/VecNormalize5 ==
  In1 : Inport
  Constant : Constant
  Demux : Demux  Outputs=[-1 1]
  Divide : Product  Inputs=*/  OutDataTypeStr=double
  Ground : Ground
  Math Function : Math  Operator=square  SignedPower=on
  Math Function1 : Math  Operator=sqrt  SignedPower=on
  Mux : Mux  Inputs=2
  Mux1 : Mux  Inputs=2
  Product : Product  RndMeth=Zero
  Sum of Elements : Sum  Inputs=+
  Switch : Switch  Criteria=u2 > Threshold  Threshold=eps  SaturateOnIntegerOverflow=off  InputSameDT=off
  Out1 : Outport  VectorParamsAs1DForOutWhenUnconnected=off
  wires:
  Math Function/1 -> Sum of Elements/1
  Demux/1 -> Divide/1
  Constant/1 -> Mux1/2
  Mux1/1 -> Switch/3
  Divide/1 -> Out1/1
  Switch/1 -> Demux/1
  Mux/1 -> Switch/1
  Demux/2 -> Divide/2
  Product/1 -> Mux1/1
  In1/1 -> Product/1, Math Function/1, Mux/1
  Ground/1 -> Product/2
  Sum of Elements/1 -> Math Function1/1
  Math Function1/1 -> Mux/2, Switch/2

== system HSat_orbit_merged_maria/Subsystem1/control/Subsystem6/Subsystem2/PPU1/VecNormalize6 ==
  In1 : Inport
  Constant : Constant
  Demux : Demux  Outputs=[-1 1]
  Divide : Product  Inputs=*/  OutDataTypeStr=double
  Ground : Ground
  Math Function : Math  Operator=square  SignedPower=on
  Math Function1 : Math  Operator=sqrt  SignedPower=on
  Mux : Mux  Inputs=2
  Mux1 : Mux  Inputs=2
  Product : Product  RndMeth=Zero
  Sum of Elements : Sum  Inputs=+
  Switch : Switch  Criteria=u2 > Threshold  Threshold=eps  SaturateOnIntegerOverflow=off  InputSameDT=off
  Out1 : Outport  VectorParamsAs1DForOutWhenUnconnected=off
  wires:
  Math Function/1 -> Sum of Elements/1
  Demux/1 -> Divide/1
  Constant/1 -> Mux1/2
  Mux1/1 -> Switch/3
  Divide/1 -> Out1/1
  Switch/1 -> Demux/1
  Mux/1 -> Switch/1
  Demux/2 -> Divide/2
  Product/1 -> Mux1/1
  In1/1 -> Product/1, Math Function/1, Mux/1
  Ground/1 -> Product/2
  Sum of Elements/1 -> Math Function1/1
  Math Function1/1 -> Mux/2, Switch/2

== system HSat_orbit_merged_maria/Subsystem1/control/Subsystem6/Subsystem2/PPU1/VecNormalize7 ==
  In1 : Inport
  Constant : Constant
  Demux : Demux  Outputs=[-1 1]
  Divide : Product  Inputs=*/  OutDataTypeStr=double
  Ground : Ground
  Math Function : Math  Operator=square  SignedPower=on
  Math Function1 : Math  Operator=sqrt  SignedPower=on
  Mux : Mux  Inputs=2
  Mux1 : Mux  Inputs=2
  Product : Product  RndMeth=Zero
  Sum of Elements : Sum  Inputs=+
  Switch : Switch  Criteria=u2 > Threshold  Threshold=eps  SaturateOnIntegerOverflow=off  InputSameDT=off
  Out1 : Outport  VectorParamsAs1DForOutWhenUnconnected=off
  wires:
  Math Function/1 -> Sum of Elements/1
  Demux/1 -> Divide/1
  Constant/1 -> Mux1/2
  Mux1/1 -> Switch/3
  Divide/1 -> Out1/1
  Switch/1 -> Demux/1
  Mux/1 -> Switch/1
  Demux/2 -> Divide/2
  Product/1 -> Mux1/1
  In1/1 -> Product/1, Math Function/1, Mux/1
  Ground/1 -> Product/2
  Sum of Elements/1 -> Math Function1/1
  Math Function1/1 -> Mux/2, Switch/2

== system HSat_orbit_merged_maria/Subsystem1/control/Subsystem6/Subsystem2/PPU1/VecNormalize8 ==
  In1 : Inport
  Constant : Constant
  Demux : Demux  Outputs=[-1 1]
  Divide : Product  Inputs=*/  OutDataTypeStr=double
  Ground : Ground
  Math Function : Math  Operator=square  SignedPower=on
  Math Function1 : Math  Operator=sqrt  SignedPower=on
  Mux : Mux  Inputs=2
  Mux1 : Mux  Inputs=2
  Product : Product  RndMeth=Zero
  Sum of Elements : Sum  Inputs=+
  Switch : Switch  Criteria=u2 > Threshold  Threshold=eps  SaturateOnIntegerOverflow=off  InputSameDT=off
  Out1 : Outport  VectorParamsAs1DForOutWhenUnconnected=off
  wires:
  Math Function/1 -> Sum of Elements/1
  Demux/1 -> Divide/1
  Constant/1 -> Mux1/2
  Mux1/1 -> Switch/3
  Divide/1 -> Out1/1
  Switch/1 -> Demux/1
  Mux/1 -> Switch/1
  Demux/2 -> Divide/2
  Product/1 -> Mux1/1
  In1/1 -> Product/1, Math Function/1, Mux/1
  Ground/1 -> Product/2
  Sum of Elements/1 -> Math Function1/1
  Math Function1/1 -> Mux/2, Switch/2

== system HSat_orbit_merged_maria/Subsystem1/control/Subsystem6/Subsystem2/PPU1+2/VecNormalize1 ==
  In1 : Inport
  Constant : Constant
  Demux : Demux  Outputs=[-1 1]
  Divide : Product  Inputs=*/  OutDataTypeStr=double
  Ground : Ground
  Math Function : Math  Operator=square  SignedPower=on
  Math Function1 : Math  Operator=sqrt  SignedPower=on
  Mux : Mux  Inputs=2
  Mux1 : Mux  Inputs=2
  Product : Product  RndMeth=Zero
  Sum of Elements : Sum  Inputs=+
  Switch : Switch  Criteria=u2 > Threshold  Threshold=eps  SaturateOnIntegerOverflow=off  InputSameDT=off
  Out1 : Outport  VectorParamsAs1DForOutWhenUnconnected=off
  wires:
  Math Function/1 -> Sum of Elements/1
  Demux/1 -> Divide/1
  Constant/1 -> Mux1/2
  Mux1/1 -> Switch/3
  Divide/1 -> Out1/1
  Switch/1 -> Demux/1
  Mux/1 -> Switch/1
  Demux/2 -> Divide/2
  Product/1 -> Mux1/1
  In1/1 -> Product/1, Math Function/1, Mux/1
  Ground/1 -> Product/2
  Sum of Elements/1 -> Math Function1/1
  Math Function1/1 -> Mux/2, Switch/2

== system HSat_orbit_merged_maria/Subsystem1/control/Subsystem6/Subsystem2/PPU1+2/VecNormalize2 ==
  In1 : Inport
  Constant : Constant
  Demux : Demux  Outputs=[-1 1]
  Divide : Product  Inputs=*/  OutDataTypeStr=double
  Ground : Ground
  Math Function : Math  Operator=square  SignedPower=on
  Math Function1 : Math  Operator=sqrt  SignedPower=on
  Mux : Mux  Inputs=2
  Mux1 : Mux  Inputs=2
  Product : Product  RndMeth=Zero
  Sum of Elements : Sum  Inputs=+
  Switch : Switch  Criteria=u2 > Threshold  Threshold=eps  SaturateOnIntegerOverflow=off  InputSameDT=off
  Out1 : Outport  VectorParamsAs1DForOutWhenUnconnected=off
  wires:
  Math Function/1 -> Sum of Elements/1
  Demux/1 -> Divide/1
  Constant/1 -> Mux1/2
  Mux1/1 -> Switch/3
  Divide/1 -> Out1/1
  Switch/1 -> Demux/1
  Mux/1 -> Switch/1
  Demux/2 -> Divide/2
  Product/1 -> Mux1/1
  In1/1 -> Product/1, Math Function/1, Mux/1
  Ground/1 -> Product/2
  Sum of Elements/1 -> Math Function1/1
  Math Function1/1 -> Mux/2, Switch/2

== system HSat_orbit_merged_maria/Subsystem1/control/Subsystem6/Subsystem2/PPU1+2/VecNormalize3 ==
  In1 : Inport
  Constant : Constant
  Demux : Demux  Outputs=[-1 1]
  Divide : Product  Inputs=*/  OutDataTypeStr=double
  Ground : Ground
  Math Function : Math  Operator=square  SignedPower=on
  Math Function1 : Math  Operator=sqrt  SignedPower=on
  Mux : Mux  Inputs=2
  Mux1 : Mux  Inputs=2
  Product : Product  RndMeth=Zero
  Sum of Elements : Sum  Inputs=+
  Switch : Switch  Criteria=u2 > Threshold  Threshold=eps  SaturateOnIntegerOverflow=off  InputSameDT=off
  Out1 : Outport  VectorParamsAs1DForOutWhenUnconnected=off
  wires:
  Math Function/1 -> Sum of Elements/1
  Demux/1 -> Divide/1
  Constant/1 -> Mux1/2
  Mux1/1 -> Switch/3
  Divide/1 -> Out1/1
  Switch/1 -> Demux/1
  Mux/1 -> Switch/1
  Demux/2 -> Divide/2
  Product/1 -> Mux1/1
  In1/1 -> Product/1, Math Function/1, Mux/1
  Ground/1 -> Product/2
  Sum of Elements/1 -> Math Function1/1
  Math Function1/1 -> Mux/2, Switch/2

== system HSat_orbit_merged_maria/Subsystem1/control/Subsystem6/Subsystem2/PPU1+2/VecNormalize4 ==
  In1 : Inport
  Constant : Constant
  Demux : Demux  Outputs=[-1 1]
  Divide : Product  Inputs=*/  OutDataTypeStr=double
  Ground : Ground
  Math Function : Math  Operator=square  SignedPower=on
  Math Function1 : Math  Operator=sqrt  SignedPower=on
  Mux : Mux  Inputs=2
  Mux1 : Mux  Inputs=2
  Product : Product  RndMeth=Zero
  Sum of Elements : Sum  Inputs=+
  Switch : Switch  Criteria=u2 > Threshold  Threshold=eps  SaturateOnIntegerOverflow=off  InputSameDT=off
  Out1 : Outport  VectorParamsAs1DForOutWhenUnconnected=off
  wires:
  Math Function/1 -> Sum of Elements/1
  Demux/1 -> Divide/1
  Constant/1 -> Mux1/2
  Mux1/1 -> Switch/3
  Divide/1 -> Out1/1
  Switch/1 -> Demux/1
  Mux/1 -> Switch/1
  Demux/2 -> Divide/2
  Product/1 -> Mux1/1
  In1/1 -> Product/1, Math Function/1, Mux/1
  Ground/1 -> Product/2
  Sum of Elements/1 -> Math Function1/1
  Math Function1/1 -> Mux/2, Switch/2

== system HSat_orbit_merged_maria/Subsystem1/control/Subsystem6/Subsystem2/PPU1+2/VecNormalize5 ==
  In1 : Inport
  Constant : Constant
  Demux : Demux  Outputs=[-1 1]
  Divide : Product  Inputs=*/  OutDataTypeStr=double
  Ground : Ground
  Math Function : Math  Operator=square  SignedPower=on
  Math Function1 : Math  Operator=sqrt  SignedPower=on
  Mux : Mux  Inputs=2
  Mux1 : Mux  Inputs=2
  Product : Product  RndMeth=Zero
  Sum of Elements : Sum  Inputs=+
  Switch : Switch  Criteria=u2 > Threshold  Threshold=eps  SaturateOnIntegerOverflow=off  InputSameDT=off
  Out1 : Outport  VectorParamsAs1DForOutWhenUnconnected=off
  wires:
  Math Function/1 -> Sum of Elements/1
  Demux/1 -> Divide/1
  Constant/1 -> Mux1/2
  Mux1/1 -> Switch/3
  Divide/1 -> Out1/1
  Switch/1 -> Demux/1
  Mux/1 -> Switch/1
  Demux/2 -> Divide/2
  Product/1 -> Mux1/1
  In1/1 -> Product/1, Math Function/1, Mux/1
  Ground/1 -> Product/2
  Sum of Elements/1 -> Math Function1/1
  Math Function1/1 -> Mux/2, Switch/2

== system HSat_orbit_merged_maria/Subsystem1/control/Subsystem6/Subsystem2/PPU1+2/VecNormalize6 ==
  In1 : Inport
  Constant : Constant
  Demux : Demux  Outputs=[-1 1]
  Divide : Product  Inputs=*/  OutDataTypeStr=double
  Ground : Ground
  Math Function : Math  Operator=square  SignedPower=on
  Math Function1 : Math  Operator=sqrt  SignedPower=on
  Mux : Mux  Inputs=2
  Mux1 : Mux  Inputs=2
  Product : Product  RndMeth=Zero
  Sum of Elements : Sum  Inputs=+
  Switch : Switch  Criteria=u2 > Threshold  Threshold=eps  SaturateOnIntegerOverflow=off  InputSameDT=off
  Out1 : Outport  VectorParamsAs1DForOutWhenUnconnected=off
  wires:
  Math Function/1 -> Sum of Elements/1
  Demux/1 -> Divide/1
  Constant/1 -> Mux1/2
  Mux1/1 -> Switch/3
  Divide/1 -> Out1/1
  Switch/1 -> Demux/1
  Mux/1 -> Switch/1
  Demux/2 -> Divide/2
  Product/1 -> Mux1/1
  In1/1 -> Product/1, Math Function/1, Mux/1
  Ground/1 -> Product/2
  Sum of Elements/1 -> Math Function1/1
  Math Function1/1 -> Mux/2, Switch/2

== system HSat_orbit_merged_maria/Subsystem1/control/Subsystem6/Subsystem2/PPU1+2/VecNormalize7 ==
  In1 : Inport
  Constant : Constant
  Demux : Demux  Outputs=[-1 1]
  Divide : Product  Inputs=*/  OutDataTypeStr=double
  Ground : Ground
  Math Function : Math  Operator=square  SignedPower=on
  Math Function1 : Math  Operator=sqrt  SignedPower=on
  Mux : Mux  Inputs=2
  Mux1 : Mux  Inputs=2
  Product : Product  RndMeth=Zero
  Sum of Elements : Sum  Inputs=+
  Switch : Switch  Criteria=u2 > Threshold  Threshold=eps  SaturateOnIntegerOverflow=off  InputSameDT=off
  Out1 : Outport  VectorParamsAs1DForOutWhenUnconnected=off
  wires:
  Math Function/1 -> Sum of Elements/1
  Demux/1 -> Divide/1
  Constant/1 -> Mux1/2
  Mux1/1 -> Switch/3
  Divide/1 -> Out1/1
  Switch/1 -> Demux/1
  Mux/1 -> Switch/1
  Demux/2 -> Divide/2
  Product/1 -> Mux1/1
  In1/1 -> Product/1, Math Function/1, Mux/1
  Ground/1 -> Product/2
  Sum of Elements/1 -> Math Function1/1
  Math Function1/1 -> Mux/2, Switch/2

== system HSat_orbit_merged_maria/Subsystem1/control/Subsystem6/Subsystem2/PPU1+2/VecNormalize8 ==
  In1 : Inport
  Constant : Constant
  Demux : Demux  Outputs=[-1 1]
  Divide : Product  Inputs=*/  OutDataTypeStr=double
  Ground : Ground
  Math Function : Math  Operator=square  SignedPower=on
  Math Function1 : Math  Operator=sqrt  SignedPower=on
  Mux : Mux  Inputs=2
  Mux1 : Mux  Inputs=2
  Product : Product  RndMeth=Zero
  Sum of Elements : Sum  Inputs=+
  Switch : Switch  Criteria=u2 > Threshold  Threshold=eps  SaturateOnIntegerOverflow=off  InputSameDT=off
  Out1 : Outport  VectorParamsAs1DForOutWhenUnconnected=off
  wires:
  Math Function/1 -> Sum of Elements/1
  Demux/1 -> Divide/1
  Constant/1 -> Mux1/2
  Mux1/1 -> Switch/3
  Divide/1 -> Out1/1
  Switch/1 -> Demux/1
  Mux/1 -> Switch/1
  Demux/2 -> Divide/2
  Product/1 -> Mux1/1
  In1/1 -> Product/1, Math Function/1, Mux/1
  Ground/1 -> Product/2
  Sum of Elements/1 -> Math Function1/1
  Math Function1/1 -> Mux/2, Switch/2

== system HSat_orbit_merged_maria/Subsystem1/control/Subsystem6/Subsystem2/PPU2/VecNormalize1 ==
  In1 : Inport
  Constant : Constant
  Demux : Demux  Outputs=[-1 1]
  Divide : Product  Inputs=*/  OutDataTypeStr=double
  Ground : Ground
  Math Function : Math  Operator=square  SignedPower=on
  Math Function1 : Math  Operator=sqrt  SignedPower=on
  Mux : Mux  Inputs=2
  Mux1 : Mux  Inputs=2
  Product : Product  RndMeth=Zero
  Sum of Elements : Sum  Inputs=+
  Switch : Switch  Criteria=u2 > Threshold  Threshold=eps  SaturateOnIntegerOverflow=off  InputSameDT=off
  Out1 : Outport  VectorParamsAs1DForOutWhenUnconnected=off
  wires:
  Math Function/1 -> Sum of Elements/1
  Demux/1 -> Divide/1
  Constant/1 -> Mux1/2
  Mux1/1 -> Switch/3
  Divide/1 -> Out1/1
  Switch/1 -> Demux/1
  Mux/1 -> Switch/1
  Demux/2 -> Divide/2
  Product/1 -> Mux1/1
  In1/1 -> Product/1, Math Function/1, Mux/1
  Ground/1 -> Product/2
  Sum of Elements/1 -> Math Function1/1
  Math Function1/1 -> Mux/2, Switch/2

== system HSat_orbit_merged_maria/Subsystem1/control/Subsystem6/Subsystem2/PPU2/VecNormalize2 ==
  In1 : Inport
  Constant : Constant
  Demux : Demux  Outputs=[-1 1]
  Divide : Product  Inputs=*/  OutDataTypeStr=double
  Ground : Ground
  Math Function : Math  Operator=square  SignedPower=on
  Math Function1 : Math  Operator=sqrt  SignedPower=on
  Mux : Mux  Inputs=2
  Mux1 : Mux  Inputs=2
  Product : Product  RndMeth=Zero
  Sum of Elements : Sum  Inputs=+
  Switch : Switch  Criteria=u2 > Threshold  Threshold=eps  SaturateOnIntegerOverflow=off  InputSameDT=off
  Out1 : Outport  VectorParamsAs1DForOutWhenUnconnected=off
  wires:
  Math Function/1 -> Sum of Elements/1
  Demux/1 -> Divide/1
  Constant/1 -> Mux1/2
  Mux1/1 -> Switch/3
  Divide/1 -> Out1/1
  Switch/1 -> Demux/1
  Mux/1 -> Switch/1
  Demux/2 -> Divide/2
  Product/1 -> Mux1/1
  In1/1 -> Product/1, Math Function/1, Mux/1
  Ground/1 -> Product/2
  Sum of Elements/1 -> Math Function1/1
  Math Function1/1 -> Mux/2, Switch/2

== system HSat_orbit_merged_maria/Subsystem1/control/Subsystem6/Subsystem2/PPU2/VecNormalize3 ==
  In1 : Inport
  Constant : Constant
  Demux : Demux  Outputs=[-1 1]
  Divide : Product  Inputs=*/  OutDataTypeStr=double
  Ground : Ground
  Math Function : Math  Operator=square  SignedPower=on
  Math Function1 : Math  Operator=sqrt  SignedPower=on
  Mux : Mux  Inputs=2
  Mux1 : Mux  Inputs=2
  Product : Product  RndMeth=Zero
  Sum of Elements : Sum  Inputs=+
  Switch : Switch  Criteria=u2 > Threshold  Threshold=eps  SaturateOnIntegerOverflow=off  InputSameDT=off
  Out1 : Outport  VectorParamsAs1DForOutWhenUnconnected=off
  wires:
  Math Function/1 -> Sum of Elements/1
  Demux/1 -> Divide/1
  Constant/1 -> Mux1/2
  Mux1/1 -> Switch/3
  Divide/1 -> Out1/1
  Switch/1 -> Demux/1
  Mux/1 -> Switch/1
  Demux/2 -> Divide/2
  Product/1 -> Mux1/1
  In1/1 -> Product/1, Math Function/1, Mux/1
  Ground/1 -> Product/2
  Sum of Elements/1 -> Math Function1/1
  Math Function1/1 -> Mux/2, Switch/2

== system HSat_orbit_merged_maria/Subsystem1/control/Subsystem6/Subsystem2/PPU2/VecNormalize4 ==
  In1 : Inport
  Constant : Constant
  Demux : Demux  Outputs=[-1 1]
  Divide : Product  Inputs=*/  OutDataTypeStr=double
  Ground : Ground
  Math Function : Math  Operator=square  SignedPower=on
  Math Function1 : Math  Operator=sqrt  SignedPower=on
  Mux : Mux  Inputs=2
  Mux1 : Mux  Inputs=2
  Product : Product  RndMeth=Zero
  Sum of Elements : Sum  Inputs=+
  Switch : Switch  Criteria=u2 > Threshold  Threshold=eps  SaturateOnIntegerOverflow=off  InputSameDT=off
  Out1 : Outport  VectorParamsAs1DForOutWhenUnconnected=off
  wires:
  Math Function/1 -> Sum of Elements/1
  Demux/1 -> Divide/1
  Constant/1 -> Mux1/2
  Mux1/1 -> Switch/3
  Divide/1 -> Out1/1
  Switch/1 -> Demux/1
  Mux/1 -> Switch/1
  Demux/2 -> Divide/2
  Product/1 -> Mux1/1
  In1/1 -> Product/1, Math Function/1, Mux/1
  Ground/1 -> Product/2
  Sum of Elements/1 -> Math Function1/1
  Math Function1/1 -> Mux/2, Switch/2
